simulink model "BodyQuarter"  (R2018b)
settings: Solver=VariableStepAuto  StartTime=0.0  StopTime=10.0  RelTol=1e-3
values from neighbouring files (symbols this model uses):
  M1 = 500    [CarQuarterParam.m]
settings Model: Creator=Reece Bell  LastModifiedBy=reece

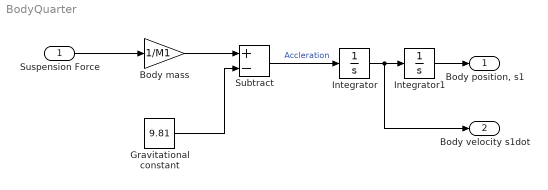
== system BodyQuarter ==
  Suspension Force : Inport
  "Body mass " : Gain  Gain=1/M1
  Gravitational constant : Constant  Value=9.81
  Integrator : Integrator
  Integrator1 : Integrator
  Subtract : Sum  Inputs=+-
  "Body position, s1" : Outport
  "Body velocity s1dot " : Outport  Port=2
  wires:
  Suspension Force/1 -> "Body mass "/1
  "Body mass "/1 -> Subtract/1
  Gravitational constant/1 -> Subtract/2
  Subtract/1 -> Integrator/1  "Accleration"
  Integrator/1 -> "Body velocity s1dot "/1, Integrator1/1
  Integrator1/1 -> "Body position, s1"/1
